simulink library "etherlab_lib"  (R2017b)
settings: Solver=ode45  StartTime=0.0  StopTime=10.0  RelTol=1e-3
undefined symbols (not defined in the file or in its folder): baumer_ecatencoder, ekxxxx, el1xxx, el2xxx, el320x_1, el331x, el3356, el3403, el36x2, el37x2, el4xxx, el500x, el5021, El5152, EL51x1, el51xx, el9xxx, ep1xxx, ep2xxx, ep41xx_1, ep8309, murr_dio
(part 1 of 4)
settings Model: ExtModeAutoUpdateStatusClock=off  Creator=rich  LastModifiedBy=ha
settings DataIOCC: LimitDataPoints=on  SaveFormat=Array  SignalLoggingSaveFormat=ModelDataLogs
settings OptimizationCC: BlockReduction=off  BooleanDataType=off  ExpressionDepthLimit=2147483647  LifeSpan=inf
settings DebuggingCC: SaveWithParameterizedLinksMsg=none  UnderspecifiedInitializationDetection=Classic  MergeDetectMultiDrivingBlocksExec=none  SignalResolutionControl=TryResolveAllWithWarning  FcnCallInpInsideContextMsg=warning  StateNameClashWarn=warning  StrictBusMsg=Warning  SFUnexpectedBacktrackingDiag=warning  SFNoUnconditionalDefaultTransitionDiag=warning  SFExecutionAtInitializationDiag=none
settings HardwareCC: ProdBitPerPointer=32  ProdBitPerSizeT=32  ProdBitPerPtrDiffT=32  ProdLargestAtomicFloat=None  ProdIntDivRoundTo=Undefined  ProdEndianess=Unspecified  ProdWordSize=32  ProdHWDeviceType=32-bit Generic  TargetUnknown=on
settings ModelReferenceCC: PropagateSignalLabelsOutOfModel=off
settings RTWCC: PostCodeGenCommand=etherlab_postprocess(modelName,buildInfo)
settings CodeAppCC: StateflowObjectComments=on
settings GRTTargetCC: TargetLangStandard=C89/C90 (ANSI)  GeneratePreprocessorConditionals=Disable all  CombineOutputUpdateFcns=off  GRTInterface=on
settings ConfigComp: CovMetricSettings=dw  CovHtmlReporting=on  CovSaveCumulativeToWorkspaceVar=on  CovSaveSingleToWorkspaceVar=on  CovExternalEMLEnable=off

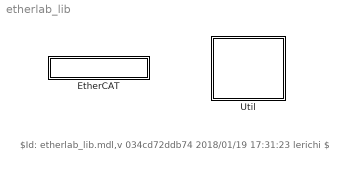
== system etherlab_lib ==
  note: $Id: etherlab_lib.mdl,v 034cd72ddb74 2018/01/19 17:31:23 lerichi $
  EtherCAT : Subsystem
      mask Display: image(imread('ethercat_mini.png'))
  Util : Subsystem
      mask Display: image(imread('tools.png'))

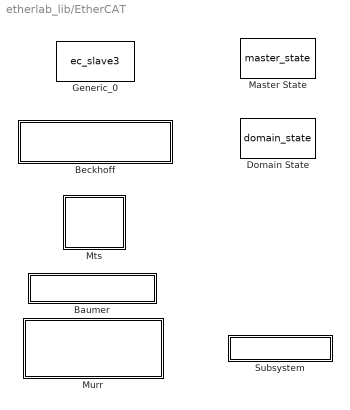
== system etherlab_lib/EtherCAT ==
  Baumer : Subsystem
      mask Display: image(imread('Baumer.png'))
  Beckhoff : Subsystem
      mask Display: image(imread('Beckhoff.png'))
  Domain State : S-Function  FunctionName=domain_state  Parameters=master,domain,input,output,io_domain,tsample  SFunctionModules='ecrt_support'  SFunctionDeploymentMode=off  EnableBusSupport=off  mask(Domain State){master=0, domain=0, direction=Input and Output, io_domain=on, tsample=0}
      mask prompts: io_domain "Tx and RxPdo in one domain"; tsample "Sample Time"
      mask help:
      | Displays the following domain state information:
      | * Working Counter
      | * Domain state:
      | 	0 - No slaves
      | 	1 - Domain incomplete
      | 	2 - Domain complete
      mask init:
      | switch direction
      |     case 1
      |         input = 1;
      |         output = 0;
      |     case 2
      |         input = 0;
      |         output = 1;
      |     case 3
      |         input = 1;
      |         output = 1;
      | end
      mask TypeOptions direction: Input Only | Output Only | Input and Output
      mask Display: fprintf('Domain State\nM:%u d:%u', master,domain);
  Generic_0 : S-Function  FunctionName=ec_slave3  Parameters=Address,rv.SlaveConfig,rv.PortConfig,debug,tsample,param  SFunctionModules='ecrt_support'  SFunctionDeploymentMode=off  EnableBusSupport=off  mask(Generic EtherCAT Slave){master=0, index=1, rv=[], param=[], tsample=0, debug=0}
      mask prompts: index "Slave Index"; rv "EtherCAT Slave Configuration struct. (SlaveConfig, PortConfig)"; param "Block Parameters"; tsample "Sample Time"
      mask help:
      | The generic EtherCAT Slave is used to create any slave not contained
      | in this library. A mask input variable, <b>EtherCAT Slave Configuration</b>,
      | has to be set up by the user. This configures the slave.
      mask init:
      | Address = EtherCATSlave.formatAddress(master,index,tsample);
      | 
      | if ~isfield(rv,'PortConfig') || isempty(rv)
      |    rv.PortConfig = [];
      | end
      | 
      | if ~isfield(rv,'SlaveConfig') || isempty(rv)
      |    rv.SlaveConfig = [];
      | end
      | 
      | if ~isfield(rv.SlaveConfig,'description') || isempty(rv)
      |    slave_name = 'unknown';
      | else
      |    slave_name = rv.SlaveConfig.description;
      | end
      mask Help: web(etherlab_help_path('generic.html'), '-helpbrowser');
      mask Display:
      | fprintf('Generic Slave\n%s \n%i Idx:%s', ...
      |     slave_name, master, mat2str(index))
  Master State : S-Function  FunctionName=master_state  Parameters=master,devices,reset,sync_dec,tsample  SFunctionModules='ecrt_support'  SFunctionDeploymentMode=off  EnableBusSupport=off  mask(Master State){master=0, devices=1, reset=off, sync_dec=0, tsample=0}
      mask prompts: devices "Device Count"; reset "Reset Port"; sync_dec "Reference Clock Sync Decimation"; tsample "Sample Time"
      mask help:
      | Outputs master state:
      | * number of responding slaves
      | * Slave states
      | * Link up
      |
      | Enabling <b>Master Reset</b> forces the master to reset the bus
      | and scan for new slaves
      mask Display: fprintf('Master State\nM: %u', master);
  Mts : Subsystem
      mask Display: image(imread('mts-logo.png'))
  Murr : Subsystem
      mask Display: image(imread('Murr.png'))
  Subsystem : Subsystem
      settings: OpenFcn=[];
      mask Display: image(imread('ethercat_mini.png'))

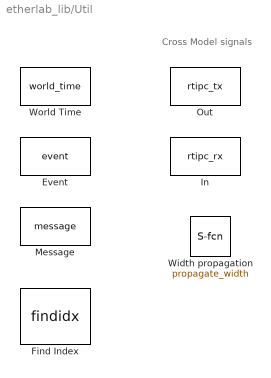
== system etherlab_lib/Util ==
  note: Cross Model signals
  Event : S-Function  FunctionName=event  Parameters=width,singleshot,dtype,tsample  SFunctionDeploymentMode=off  EnableBusSupport=off  mask(Trigger Events){width=-1, singleshot=on, dtype_str=Boolean, tsample=eval(get_param(bdroot,'FixedStep'))}
      mask prompts: singleshot "Single shot"; dtype_str "Data Type"; tsample "Sample Time"
      mask help:
      | This block is used to generate an events on its output.
      |
      | Checking the "One Shot" option will generate only one event, otherwise a whole chain of events is generated for every count that the parameter value was incremented.
      |
      | Width specifies output port width. If -1 is chosen, an input port appears, propagating the width to the output.
      mask init:
      | switch dtype_str
      |     case 'Unsigned Integer'
      |         dtype = 32;
      |     case 'Boolean'
      |         dtype = 1;
      |     case 'Dynamically Typed';
      |         dtype = -1;
      |     otherwise
      |         dtype = 1;
      | end
      mask Help:
      | A typical problem with interactive constants, e.g. those that are connected to push buttons on the desktop, is that the events get lost due to it being set and reset too within one calculation cycle and thus is "lost".
      | 
      | This typically happens with push buttons acting on a constant. Sometimes the user presses and releases the push button so quickly that these separate events are send to the Real Time Application together as a single operation. The constant is then set and reset without the Application realising that there even was an event.
      | 
      | This block is overcomes this limitation by keeping an internal counter synchronised to a parameter value. If these two values are unequal, the output is toggled either:
      | * If the "Single Shot" option is checked, only one event pulse is generated and the internal counter is set to the parameter value.
      | * Without this option, the internal counter is incremented until it equals the parameter value, generating one event pulse for every increment.
      mask TypeOptions dtype_str: Boolean | Unsigned Integer | Dynamically Typed
      mask Display: disp('Event')
  Find Index : S-Function  FunctionName=findidx  Parameters=cmp,tsample  SFunctionDeploymentMode=off  EnableBusSupport=off  mask(Find MinMax){cmp=First Minimum, tsample=-1}
      mask prompts: cmp "Comparison"; tsample "Sample Time"
      mask help:
      | This block takes a vector input and outputs:
      | 1: Found count
      | 2: Found Index (zero based)
      | 3: Value
      mask Help: This block finds the minimum or or maximum as well as the associated index from a vector of signals. The index is zero based.
      mask TypeOptions cmp: First Minimum | Last Minimum | First Maximum | Last Maximum
      mask Display:
      | port_label('output',1,'Found');
      | port_label('output',2,'Index');
      | port_label('output',3,'Value');
  In : S-Function  FunctionName=rtipc_rx  Parameters=varname,dtype,len,force,tsample  SFunctionModules='rtipc'  SFunctionDeploymentMode=off  EnableBusSupport=off  mask(Generic Output Port){varname='SIG01', dtype=double, len=1, force=off, tsample=0}
      mask prompts: varname "Signal Name"; dtype "Data Type"; len "Vector Length"; force "Enable value forcing"; tsample "Sample Time (-1 for inherited)"
      mask help:
      | RealTime Interprocess Communication input
      |
      | Signal Name: Name of signal to connect to (string)
      | Data Type: Signal's data type
      | Vector Length: Number of elements
      | Enable Force Value: Adds additional parameters to force the output value
      mask TypeOptions dtype: boolean | int8 | uint8 | int16 | uint16 | int32 | uint32 | single | double
      mask Display: fprintf(varname)
  Message : S-Function  FunctionName=message  Parameters=prio,message_text,reset,invert,confirm,tsample  SFunctionDeploymentMode=off  EnableBusSupport=off  mask(Generate system message){prio=Error, message_text={}, reset=on, invert=off, confirm=[], tsample=-1}
      mask prompts: prio "Priority"; message_text "Message List"; reset "External Reset"; invert "Invert Input"; confirm "Input confirm delay [s]"; tsample "Sample Time (-1 for inherited)"
      mask help:
      | This block generates a system message when the input port 1 is true.
      |
      | The current time is output on output port.
      mask init:
      | m = {'Emergency', 'Alert', 'Critical', 'Error', ...
      |     'Warning', 'Notice', 'Information', 'Debug'};
      | cmap = [
      |     1 0 1;
      |     1 0 1;
      |     1 0 1;
      |     1 0 0;
      |     1 0.5 0.0;
      |     0 0 1;
      |     0 0 1;
      |     0 0 1;
      |     ]; 
      | c = cmap(prio,:);
      | priority = m{prio};
      mask Help:
      | This block generates a system message when the input port 1 is true.
      | System messages are logged and kept in history.
      | 
      | <h2>Parameters:</h2>
      | 
      | <h4>Priority</h4>Select the message priority
      | 
      | <h4>Message List</h4> Enter the message to be printed.
      | It must be a cell array of strings and have the same number of
      | elements as port 1.
      | 
      | <h4>External Reset</h4>Message will be reset on external signal.
      | 
      | <h4>Invert Input</h4>Invert input (0 = Generate message)
      | 
      | <h4>Input confirm delay</h4>Delay time before message is raised.
      mask TypeOptions prio: Emergency | Alert | Critical | Error | Warning | Notice | Information | Debug
      mask Display:
      | patch([0,0,1,1],[0,1,1,0],c);
      | disp(priority);
  Out : S-Function  FunctionName=rtipc_tx  Parameters=varname,force,tsample  SFunctionModules='rtipc'  SFunctionDeploymentMode=off  EnableBusSupport=off  mask(Generic Output Port){varname='SIG01', force=off, tsample=-1}
      mask prompts: varname "Signal Name"; force "Enable value forcing"; tsample "Sample Time (-1 for inherited)"
      mask Display: fprintf(varname)
  Width propagation : S-Function  FunctionName=propagate_width  Parameters=count,width  SFunctionDeploymentMode=off  EnableBusSupport=off  mask(Propagate width){count=2, width=-1}
      mask prompts: count "Port Count"; width "Width (-1 = inherited)"
      mask help:
      | This block forces all input ports to have the same width
      | if width is a positive integer, otherwise the width of
      | port 1 is propagated to all ports.
      mask init:
      | if width <= 0
      |     width = -1;
      |     widthstr = '=';
      | else
      |     widthstr = num2str(width);
      | end
      mask Display:
      | plot([0.05,0.95;0.3,0.7]',[0.5,0.5;0.3,0.7]')
      | text(0.5,0.8,widthstr)
  World Time : S-Function  FunctionName=world_time  Parameters=tsample  SFunctionDeploymentMode=off  EnableBusSupport=off  mask(World Time){tsample=0}
      mask prompts: tsample "Sample Time"
      mask help: Outputs the current world time for the given sample time.
      mask Help: This block outputs the hosts current real world time in seconds since 1.1.1970

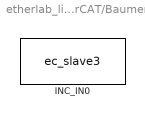
== system etherlab_lib/EtherCAT/Baumer ==
  INC_IN0 : S-Function  LoadFcn=baumer_ecatencoder().checkModelName  FunctionName=ec_slave3  Parameters=Address,rv.SlaveConfig,rv.PortConfig,debug,tsample  SFunctionModules='ecrt_support'  SFunctionDeploymentMode=off  EnableBusSupport=off  mask(Baumer && Thalheim ATD Encoder){master=0, index=1, model=BT ATD4, revision=[1 2], direction=CW, tsample=0, debug=, dc_mode=Free Run/SM-Synchron, dc_assign_activate=, dc_cycle0=[], dc_cycle0_factor=[], dc_shift0=[], dc_shift0_factor=[], dc_shift0_input=off, dc_cycle1=[], dc_cycle1_factor=[], dc_shift1=[], dc_shift1_factor=[]}
      mask prompts: index "Slave Index"; model "Device Model"; direction "Counting direction"; tsample "Sample Time (-1 for inherited)"; dc_mode "Mode"; dc_assign_activate "Assign Activate"; dc_cycle0 "Cycle Time Sync 0"; dc_cycle0_factor "Factor"; dc_shift0 "Shift Time Sync0"; dc_shift0_factor "Factor"; dc_shift0_input "Shift Time0 Input"; dc_cycle1 "Cycle Time Sync1"; dc_cycle1_factor "Factor"; dc_shift1 "Shift Time Sync1"; dc_shift1_factor "Factor"
      mask help: Baumer & Thalheim ATD Encoder
      mask init:
      | Address = EtherCATSlave.formatAddress(master,index,tsample);
      | 
      | rv = baumer_ecatencoder(model).configure(direction-1,...
      |     [dc_mode, dc_assign_activate, ...
      |      dc_cycle0, dc_cycle0_factor, ...
      |      dc_shift0, dc_shift0_factor, dc_shift0_input, ...
      |      dc_cycle1, dc_cycle1_factor, ...
      |      dc_shift1, dc_shift1_factor]);
      mask Help: web(etherlab_help_path('baumer-ecatencoder.html'), '-helpbrowser');
      mask TypeOptions model: BT ATD4 | BT ATD2 | BT ATD2_PoE
      mask Callback model: baumer_ecatencoder.modelChanged
      mask TypeOptions direction: CW | CCW
      mask TypeOptions dc_mode: Free Run/SM-Synchron | DC-Synchron | Custom
      mask Callback dc_mode: EtherCATSlave.updateCustomDCEnable()
      mask Display: fprintf('%s\nM:%i Idx:%s',model,master,mat2str(index))
